simulink model "requirement_table_only"  (R2022b)
settings: Solver=FixedStepAuto  StartTime=0.0  StopTime=10.0  FixedStep=1e-3  RelTol=1e-3  EnableMultiTasking=on
settings Model: ExtModeTrigDuration=5  Creator=dinghao  LastModifiedBy=dinghao
settings SolverCC: AlgebraicLoopSolver=TrustRegion
settings OptimizationCC: EnhancedBackFolding=on  PassReuseOutputArgsAs=Individual arguments  ZeroExternalMemoryAtStartup=off  ZeroInternalMemoryAtStartup=off  MaxStackSize=64  OptimizeBlockOrder=speed  DifferentSizesBufferReuse=on  OptimizationCustomize=off  EfficientTunableParamExpr=on
settings DebuggingCC: ParameterTunabilityLossMsg=error  UnconnectedInputMsg=warning  UnconnectedOutputMsg=warning  UnconnectedLineMsg=warning  SFMachineParentedDataDiag=warning
settings HardwareCC: ProdBitPerPointer=32  ProdBitPerSizeT=32  ProdBitPerPtrDiffT=32  ProdLargestAtomicInteger=Long  ProdLargestAtomicFloat=Double  ProdWordSize=32  ProdHWDeviceType=ARM Compatible->ARM Cortex
settings ModelReferenceCC: EnableRefExpFcnMdlSchedulingChecks=on
settings SFSimCC: MATLABDynamicMemAlloc=off
settings RTWCC: Description=Embedded Coder  SystemTargetFile=ert.tlc  HardwareBoard=NXP FRDM-K64F  TLCOptions="-aInlineSetEventsForThisBaseRateFcn=TLC_FALSE -aSuppressMultiTaskScheduler=TLC_FALSE  -aRateBasedStepFcn=0"  TemplateMakefile=ert_default_tmf  Toolchain=GNU Tools for ARM Embedded Processors
settings CodeAppCC: ForceParamTrailComments=on  IgnoreCustomStorageClasses=off  OperatorAnnotations=on  SimulinkDataObjDesc=on  SFDataObjDesc=on  InsertBlockDesc=on

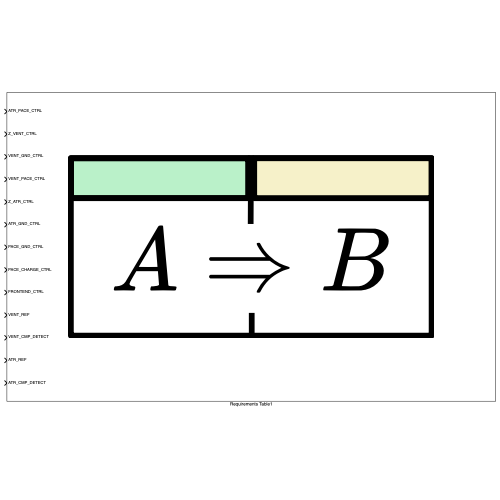
[thumbnail: Simulink's stored preview of the top-level diagram]
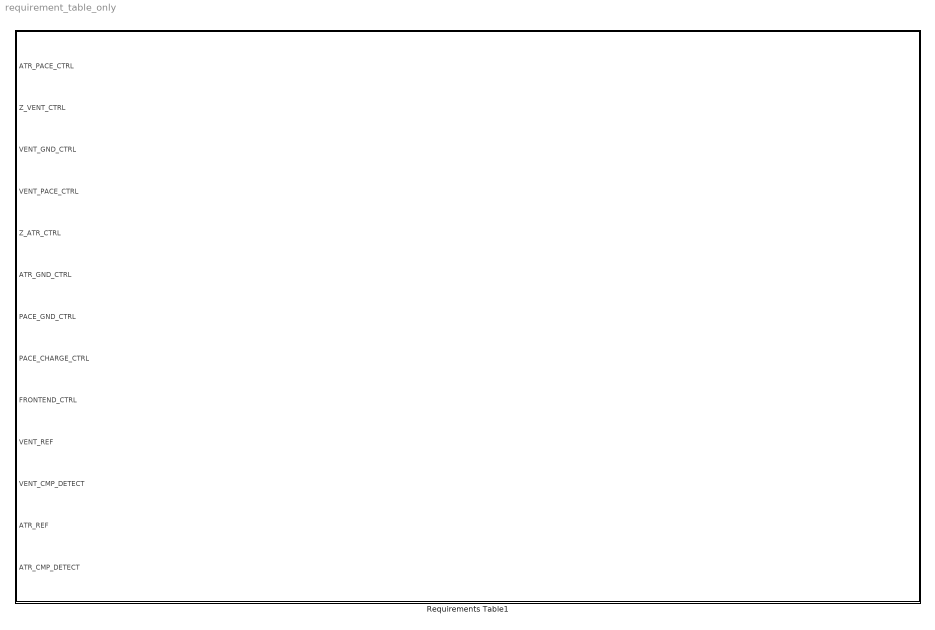
== system requirement_table_only ==
  Requirements Table1 : Requirements Table  TreatAsAtomicUnit=on

== stateflow chart requirement_table_only/Requirements Table1 ==
  (default) -> (junction 1073753366)
  (junction 1073753366) -> (junction 1073753367) : {
      | % SF_REQ_REV_07
      | }
  (junction 1073753367) -> (junction 1073753369) : {
      | % HEADER_ASSIGNMENTS
      |
      | }
  (junction 1073753369) -> (junction 1073753371) : {
      | % START_A_4
      | }
  (junction 1073753371) -> (junction 1073753373) : {
      | }
  (junction 1073753373) -> (junction 1073753375)
  (junction 1073753375) -> (junction 1073753377) : {
      | }
  (junction 1073753377) -> (junction 1073753379) : {
      | % END_A_4
      | }
  (junction 1073753379) -> (junction 1073753381) : {
      | % START_R_1
      | }
  (junction 1073753381) -> (junction 1073753383) : {
      | }
  (junction 1073753383) -> (junction 1073753385) : {
      |
      |
      |
      |
      |
      |
      |
      | }
  (junction 1073753385) -> (junction 1073753387) : {
      | }
  (junction 1073753387) -> (junction 1073753389) : {
      | % START_R_10
      | }
  (junction 1073753389) -> (junction 1073753391) : {
      | }
  (junction 1073753391) -> (junction 1073753393)
  (junction 1073753393) -> (junction 1073753395) [order 1] : [duration((prev(ATR_PACE_CTRL) == false) && (prev(PACE_CHARGE_CTRL) == true) && (prev(PACE_GND_CTRL) == true) && (prev(ATR_GND_CTRL) == true) && (prev(Z_ATR_CTRL) == false)) >= 60000/LRL-ATR_PULSE_WIDTH]
  (junction 1073753393) -> (junction 1073753401) [order 2]
  (junction 1073753395) -> (junction 1073753397) : {
      | ATR_PACE_CTRL == true
      | PACE_CHARGE_CTRL == false
      | PACE_GND_CTRL == true
      | ATR_GND_CTRL == false
      | Z_ATR_CTRL == false
      |
      |
      | }
  (junction 1073753397) -> (junction 1073753399) : {
      | }
  (junction 1073753399) -> (junction 1073753401)
  (junction 1073753401) -> (junction 1073753403)
  (junction 1073753403) -> (junction 1073753405) : {
      | % END_R_10
      | }
  (junction 1073753405) -> (junction 1073753407) : {
      | % START_R_13
      | }
  (junction 1073753407) -> (junction 1073753409) : {
      | }
  (junction 1073753409) -> (junction 1073753411)
  (junction 1073753411) -> (junction 1073753413) [order 1] : [duration((prev(ATR_PACE_CTRL) == true) && (prev(PACE_CHARGE_CTRL)== false) && (prev(PACE_GND_CTRL) == true) && (prev(ATR_GND_CTRL) == false) && (prev(Z_ATR_CTRL) == false)) >= ATR_PULSE_WIDTH]
  (junction 1073753411) -> (junction 1073753419) [order 2]
  (junction 1073753413) -> (junction 1073753415) : {
      | ATR_PACE_CTRL == false
      | PACE_CHARGE_CTRL == true
      | PACE_GND_CTRL == true
      | ATR_GND_CTRL == true
      | Z_ATR_CTRL == false
      |
      |
      | }
  (junction 1073753415) -> (junction 1073753417) : {
      | }
  (junction 1073753417) -> (junction 1073753419)
  (junction 1073753419) -> (junction 1073753421)
  (junction 1073753421) -> (junction 1073753423) : {
      | % END_R_13
      | }
  (junction 1073753423) -> (junction 1073753425) : {
      | % END_R_1
      | }
  (junction 1073753425) -> (junction 1073753427) : {
      | % START_R_16
      | }
  (junction 1073753427) -> (junction 1073753429) : {
      | }
  (junction 1073753429) -> (junction 1073753431) : {
      |
      |
      |
      |
      |
      |
      |
      | }
  (junction 1073753431) -> (junction 1073753433) : {
      | }
  (junction 1073753433) -> (junction 1073753435) : {
      | % START_R_19
      | }
  (junction 1073753435) -> (junction 1073753437) : {
      | }
  (junction 1073753437) -> (junction 1073753439)
  (junction 1073753439) -> (junction 1073753441) [order 1] : [duration((prev(VENT_PACE_CTRL) == false) && (prev(PACE_CHARGE_CTRL) == true) && (prev(VENT_GND_CTRL) == true) && (prev(PACE_GND_CTRL) == true) && (prev(Z_VENT_CTRL) == false)) >= 60000/LRL-VENT_PULSE_WIDTH]
  (junction 1073753439) -> (junction 1073753447) [order 2]
  (junction 1073753441) -> (junction 1073753443) : {
      | VENT_PACE_CTRL == true
      | PACE_CHARGE_CTRL == false
      | VENT_GND_CTRL == false
      | PACE_GND_CTRL == true
      | Z_VENT_CTRL == false
      |
      |
      | }
  (junction 1073753443) -> (junction 1073753445) : {
      | }
  (junction 1073753445) -> (junction 1073753447)
  (junction 1073753447) -> (junction 1073753449)
  (junction 1073753449) -> (junction 1073753451) : {
      | % END_R_19
      | }
  (junction 1073753451) -> (junction 1073753453) : {
      | % START_R_22
      | }
  (junction 1073753453) -> (junction 1073753455) : {
      | }
  (junction 1073753455) -> (junction 1073753457)
  (junction 1073753457) -> (junction 1073753459) [order 1] : [duration((prev(VENT_PACE_CTRL) == true) && (prev(PACE_CHARGE_CTRL) == false) && (prev(VENT_GND_CTRL) == false) && (prev(PACE_GND_CTRL) == true) && (prev(Z_VENT_CTRL) == false)) >= VENT_PULSE_WIDTH]
  (junction 1073753457) -> (junction 1073753465) [order 2]
  (junction 1073753459) -> (junction 1073753461) : {
      | VENT_PACE_CTRL == false
      | PACE_CHARGE_CTRL == true
      | VENT_GND_CTRL == true
      | PACE_GND_CTRL == true
      | Z_VENT_CTRL == false
      |
      |
      | }
  (junction 1073753461) -> (junction 1073753463) : {
      | }
  (junction 1073753463) -> (junction 1073753465)
  (junction 1073753465) -> (junction 1073753467)
  (junction 1073753467) -> (junction 1073753469) : {
      | % END_R_22
      | }
  (junction 1073753469) -> (junction 1073753471) : {
      | % END_R_16
      | }
  (junction 1073753471) -> (junction 1073753473) : {
      | % START_R_25
      | }
  (junction 1073753473) -> (junction 1073753475) : {
      | }
  (junction 1073753475) -> (junction 1073753477) : {
      |
      |
      |
      |
      |
      |
      |
      | }
  (junction 1073753477) -> (junction 1073753479) : {
      | }
  (junction 1073753479) -> (junction 1073753481) : {
      | % START_R_28
      | }
  (junction 1073753481) -> (junction 1073753483) : {
      | }
  (junction 1073753483) -> (junction 1073753485)
  (junction 1073753485) -> (junction 1073753487) [order 1] : [(prev(FRONTEND_CTRL) == true ) && (prev(VENT_PACE_CTRL) == false) && (prev(PACE_CHARGE_CTRL) == true) && (prev(PACE_GND_CTRL) == true) && (prev(VENT_GND_CTRL) == true) && (prev(Z_VENT_CTRL) == false)]
  (junction 1073753485) -> (junction 1073753529) [order 2]
  (junction 1073753487) -> (junction 1073753489) : {
      |
      |
      |
      |
      |
      |
      |
      | }
  (junction 1073753489) -> (junction 1073753491) : {
      | }
  (junction 1073753491) -> (junction 1073753493) : {
      | % START_R_49
      | }
  (junction 1073753493) -> (junction 1073753495) : {
      | }
  (junction 1073753495) -> (junction 1073753497)
  (junction 1073753497) -> (junction 1073753499) [order 1] : [(prev(VENT_CMP_DETECT) == true)]
  (junction 1073753497) -> (junction 1073753505) [order 2]
  (junction 1073753499) -> (junction 1073753501) : {
      | (FRONTEND_CTRL) == false
      | (VENT_PACE_CTRL) == false
      | (PACE_CHARGE_CTRL) == true
      | (PACE_GND_CTRL) == true
      | (VENT_GND_CTRL) == true
      | (Z_VENT_CTRL) == false
      |
      | }
  (junction 1073753501) -> (junction 1073753503) : {
      | }
  (junction 1073753503) -> (junction 1073753505)
  (junction 1073753505) -> (junction 1073753507)
  (junction 1073753507) -> (junction 1073753509) : {
      | % END_R_49
      | }
  (junction 1073753509) -> (junction 1073753511) : {
      | % START_R_52
      | }
  (junction 1073753511) -> (junction 1073753513) : {
      | }
  (junction 1073753513) -> (junction 1073753515)
  (junction 1073753515) -> (junction 1073753517) [order 1] : [duration((prev(VENT_CMP_DETECT) == false)) >= 60000/LRL-VENT_PULSE_WIDTH]
  (junction 1073753515) -> (junction 1073753523) [order 2]
  (junction 1073753517) -> (junction 1073753519) : {
      | (FRONTEND_CTRL) == true
      | (VENT_PACE_CTRL) == true
      | (PACE_CHARGE_CTRL) == false
      | (PACE_GND_CTRL) == true
      | (VENT_GND_CTRL) == false
      | (Z_VENT_CTRL) == false
      |
      | }
  (junction 1073753519) -> (junction 1073753521) : {
      | }
  (junction 1073753521) -> (junction 1073753523)
  (junction 1073753523) -> (junction 1073753525)
  (junction 1073753525) -> (junction 1073753527) : {
      | % END_R_52
      | }
  (junction 1073753527) -> (junction 1073753529)
  (junction 1073753529) -> (junction 1073753531)
  (junction 1073753531) -> (junction 1073753533) : {
      | % END_R_28
      | }
  (junction 1073753533) -> (junction 1073753535) : {
      | % START_R_31
      | }
  (junction 1073753535) -> (junction 1073753537) : {
      | }
  (junction 1073753537) -> (junction 1073753539)
  (junction 1073753539) -> (junction 1073753541) [order 1] : [duration((prev(FRONTEND_CTRL) == true ) && (prev(VENT_PACE_CTRL) == true) && (prev(PACE_CHARGE_CTRL) == false) && (prev(PACE_GND_CTRL) == true) && (prev(VENT_GND_CTRL) == false) && (prev(Z_VENT_CTRL) == false)) >= VENT_PULSE_WIDTH]
  (junction 1073753539) -> (junction 1073753583) [order 2]
  (junction 1073753541) -> (junction 1073753543) : {
      |
      |
      |
      |
      |
      |
      |
      | }
  (junction 1073753543) -> (junction 1073753545) : {
      | }
  (junction 1073753545) -> (junction 1073753547) : {
      | % START_R_55
      | }
  (junction 1073753547) -> (junction 1073753549) : {
      | }
  (junction 1073753549) -> (junction 1073753551)
  (junction 1073753551) -> (junction 1073753553) [order 1] : [(prev(VENT_CMP_DETECT) == true)]
  (junction 1073753551) -> (junction 1073753559) [order 2]
  (junction 1073753553) -> (junction 1073753555) : {
      | (FRONTEND_CTRL) == false
      | (VENT_PACE_CTRL) == false
      | (PACE_CHARGE_CTRL) == true
      | (PACE_GND_CTRL) == true
      | (VENT_GND_CTRL) == true
      | (Z_VENT_CTRL) == false
      |
      | }
  (junction 1073753555) -> (junction 1073753557) : {
      | }
  (junction 1073753557) -> (junction 1073753559)
  (junction 1073753559) -> (junction 1073753561)
  (junction 1073753561) -> (junction 1073753563) : {
      | % END_R_55
      | }
  (junction 1073753563) -> (junction 1073753565) : {
      | % START_R_58
      | }
  (junction 1073753565) -> (junction 1073753567) : {
      | }
  (junction 1073753567) -> (junction 1073753569)
  (junction 1073753569) -> (junction 1073753571) [order 1] : [(prev(VENT_CMP_DETECT) == false)]
  (junction 1073753569) -> (junction 1073753577) [order 2]
  (junction 1073753571) -> (junction 1073753573) : {
      | (FRONTEND_CTRL) == true
      | (VENT_PACE_CTRL) == false
      | (PACE_CHARGE_CTRL) == true
      | (PACE_GND_CTRL) == true
      | (VENT_GND_CTRL) == true
      | (Z_VENT_CTRL) == false
      |
      | }
  (junction 1073753573) -> (junction 1073753575) : {
      | }
  (junction 1073753575) -> (junction 1073753577)
  (junction 1073753577) -> (junction 1073753579)
  (junction 1073753579) -> (junction 1073753581) : {
      | % END_R_58
      | }
  (junction 1073753581) -> (junction 1073753583)
  (junction 1073753583) -> (junction 1073753585)
  (junction 1073753585) -> (junction 1073753587) : {
      | % END_R_31
      | }
  (junction 1073753587) -> (junction 1073753589) : {
      | % START_R_34
      | }
  (junction 1073753589) -> (junction 1073753591) : {
      | }
  (junction 1073753591) -> (junction 1073753593)
  (junction 1073753593) -> (junction 1073753595) [order 1] : [(prev(FRONTEND_CTRL) == false) && (prev(VENT_PACE_CTRL) == false) && (prev(PACE_CHARGE_CTRL) == true) && (prev(PACE_GND_CTRL) == true) && (prev(VENT_GND_CTRL) == true) && (prev(Z_VENT_CTRL) == false)]
  (junction 1073753593) -> (junction 1073753601) [order 2]
  (junction 1073753595) -> (junction 1073753597) : {
      | (FRONTEND_CTRL) == true
      | (VENT_PACE_CTRL) == false
      | (PACE_CHARGE_CTRL) == true
      | (PACE_GND_CTRL) == true
      | (VENT_GND_CTRL) == true
      | (Z_VENT_CTRL) == false
      |
      | }
  (junction 1073753597) -> (junction 1073753599) : {
      | }
  (junction 1073753599) -> (junction 1073753601)
  (junction 1073753601) -> (junction 1073753603)
  (junction 1073753603) -> (junction 1073753605) : {
      | % END_R_34
      | }
  (junction 1073753605) -> (junction 1073753607) : {
      | % END_R_25
      | }
  (junction 1073753607) -> (junction 1073753609) : {
      | % START_R_37
      | }
  (junction 1073753609) -> (junction 1073753611) : {
      | }
  (junction 1073753611) -> (junction 1073753613) : {
      |
      |
      |
      |
      |
      |
      |
      | }
  (junction 1073753613) -> (junction 1073753615) : {
      | }
  (junction 1073753615) -> (junction 1073753617) : {
      | % START_R_40
      | }
  (junction 1073753617) -> (junction 1073753619) : {
      | }
  (junction 1073753619) -> (junction 1073753621)
  (junction 1073753621) -> (junction 1073753623) [order 1] : [(prev(FRONTEND_CTRL) == true ) && (prev(ATR_PACE_CTRL) == false) && (prev(PACE_CHARGE_CTRL) == true) && (prev(PACE_GND_CTRL) == true) && (prev(ATR_GND_CTRL) == true) && (prev(Z_ATR_CTRL) == false)]
  (junction 1073753621) -> (junction 1073753665) [order 2]
  (junction 1073753623) -> (junction 1073753625) : {
      |
      |
      |
      |
      |
      |
      |
      | }
  (junction 1073753625) -> (junction 1073753627) : {
      | }
  (junction 1073753627) -> (junction 1073753629) : {
      | % START_R_61
      | }
  (junction 1073753629) -> (junction 1073753631) : {
      | }
  (junction 1073753631) -> (junction 1073753633)
  (junction 1073753633) -> (junction 1073753635) [order 1] : [(prev(ATR_CMP_DETECT) == true)]
  (junction 1073753633) -> (junction 1073753641) [order 2]
  (junction 1073753635) -> (junction 1073753637) : {
      | (FRONTEND_CTRL) == false
      | (ATR_PACE_CTRL) == false
      | (PACE_CHARGE_CTRL) == true
      | (PACE_GND_CTRL) == true
      | (ATR_GND_CTRL) == true
      | (Z_ATR_CTRL) == false
      |
      | }
  (junction 1073753637) -> (junction 1073753639) : {
      | }
  (junction 1073753639) -> (junction 1073753641)
  (junction 1073753641) -> (junction 1073753643)
  (junction 1073753643) -> (junction 1073753645) : {
      | % END_R_61
      | }
  (junction 1073753645) -> (junction 1073753647) : {
      | % START_R_64
      | }
  (junction 1073753647) -> (junction 1073753649) : {
      | }
  (junction 1073753649) -> (junction 1073753651)
  (junction 1073753651) -> (junction 1073753653) [order 1] : [duration((prev(ATR_CMP_DETECT) == false)) >= 60000/LRL-ATR_PULSE_WIDTH]
  (junction 1073753651) -> (junction 1073753659) [order 2]
  (junction 1073753653) -> (junction 1073753655) : {
      | (FRONTEND_CTRL) == true
      | (ATR_PACE_CTRL) == true
      | (PACE_CHARGE_CTRL) == false
      | (PACE_GND_CTRL) == true
      | (ATR_GND_CTRL) == false
      | (Z_ATR_CTRL) == false
      |
      | }
  (junction 1073753655) -> (junction 1073753657) : {
      | }
  (junction 1073753657) -> (junction 1073753659)
  (junction 1073753659) -> (junction 1073753661)
  (junction 1073753661) -> (junction 1073753663) : {
      | % END_R_64
      | }
  (junction 1073753663) -> (junction 1073753665)
  (junction 1073753665) -> (junction 1073753667)
  (junction 1073753667) -> (junction 1073753669) : {
      | % END_R_40
      | }
  (junction 1073753669) -> (junction 1073753671) : {
      | % START_R_43
      | }
  (junction 1073753671) -> (junction 1073753673) : {
      | }
  (junction 1073753673) -> (junction 1073753675)
  (junction 1073753675) -> (junction 1073753677) [order 1] : [duration((prev(FRONTEND_CTRL) == true ) && (prev(ATR_PACE_CTRL) == true) && (prev(PACE_CHARGE_CTRL) == false) && (prev(PACE_GND_CTRL) == true) && (prev(ATR_GND_CTRL) == false) && (prev(Z_ATR_CTRL) == false)) >= ATR_PULSE_WIDTH]
  (junction 1073753675) -> (junction 1073753719) [order 2]
  (junction 1073753677) -> (junction 1073753679) : {
      |
      |
      |
      |
      |
      |
      |
      | }
  (junction 1073753679) -> (junction 1073753681) : {
      | }
  (junction 1073753681) -> (junction 1073753683) : {
      | % START_R_67
      | }
  (junction 1073753683) -> (junction 1073753685) : {
      | }
  (junction 1073753685) -> (junction 1073753687)
  (junction 1073753687) -> (junction 1073753689) [order 1] : [(prev(VENT_CMP_DETECT) == true)]
  (junction 1073753687) -> (junction 1073753695) [order 2]
  (junction 1073753689) -> (junction 1073753691) : {
      | (FRONTEND_CTRL) == false
      | (ATR_PACE_CTRL) == false
      | (PACE_CHARGE_CTRL) == true
      | (PACE_GND_CTRL) == true
      | (ATR_GND_CTRL) == true
      | (Z_ATR_CTRL) == false
      |
      | }
  (junction 1073753691) -> (junction 1073753693) : {
      | }
  (junction 1073753693) -> (junction 1073753695)
  (junction 1073753695) -> (junction 1073753697)
  (junction 1073753697) -> (junction 1073753699) : {
      | % END_R_67
      | }
  (junction 1073753699) -> (junction 1073753701) : {
      | % START_R_70
      | }
  (junction 1073753701) -> (junction 1073753703) : {
      | }
  (junction 1073753703) -> (junction 1073753705)
  (junction 1073753705) -> (junction 1073753707) [order 1] : [(prev(VENT_CMP_DETECT) == false)]
  (junction 1073753705) -> (junction 1073753713) [order 2]
  (junction 1073753707) -> (junction 1073753709) : {
      | (FRONTEND_CTRL) == true
      | (ATR_PACE_CTRL) == false
      | (PACE_CHARGE_CTRL) == true
      | (PACE_GND_CTRL) == true
      | (ATR_GND_CTRL) == true
      | (Z_ATR_CTRL) == false
      |
      | }
  (junction 1073753709) -> (junction 1073753711) : {
      | }
  (junction 1073753711) -> (junction 1073753713)
  (junction 1073753713) -> (junction 1073753715)
  (junction 1073753715) -> (junction 1073753717) : {
      | % END_R_70
      | }
  (junction 1073753717) -> (junction 1073753719)
  (junction 1073753719) -> (junction 1073753721)
  (junction 1073753721) -> (junction 1073753723) : {
      | % END_R_43
      | }
  (junction 1073753723) -> (junction 1073753725) : {
      | % START_R_46
      | }
  (junction 1073753725) -> (junction 1073753727) : {
      | }
  (junction 1073753727) -> (junction 1073753729)
  (junction 1073753729) -> (junction 1073753731) [order 1] : [(prev(FRONTEND_CTRL) == false) && (prev(ATR_PACE_CTRL) == false) && (prev(PACE_CHARGE_CTRL) == true) && (prev(PACE_GND_CTRL) == true) && (prev(ATR_GND_CTRL) == true) && (prev(Z_ATR_CTRL) == false)]
  (junction 1073753729) -> (junction 1073753737) [order 2]
  (junction 1073753731) -> (junction 1073753733) : {
      | (FRONTEND_CTRL) == true
      | (ATR_PACE_CTRL) == false
      | (PACE_CHARGE_CTRL) == true
      | (PACE_GND_CTRL) == true
      | (ATR_GND_CTRL) == true
      | (Z_ATR_CTRL) == false
      |
      | }
  (junction 1073753733) -> (junction 1073753735) : {
      | }
  (junction 1073753735) -> (junction 1073753737)
  (junction 1073753737) -> (junction 1073753739)
  (junction 1073753739) -> (junction 1073753741) : {
      | % END_R_46
      | }
  (junction 1073753741) -> (junction 1073753743) : {
      | % END_R_37
      | }
  data: ATR_PACE_CTRL input boolean; Z_VENT_CTRL input boolean; VENT_GND_CTRL input boolean; VENT_PACE_CTRL input boolean; Z_ATR_CTRL input boolean; ATR_GND_CTRL input boolean; PACE_GND_CTRL input boolean; PACE_CHARGE_CTRL input boolean; FRONTEND_CTRL input boolean; VENT_REF input int8; VENT_CMP_DETECT input boolean; ATR_REF input int8; LRL constant int8; VENT_PULSE_WIDTH constant int8; ATR_PULSE_WIDTH constant int8; ATR_CMP_DETECT input boolean
